simulink model "model_bicycle"  (R2024b)
settings: Solver=ode8  StartTime=0.0  StopTime=T  FixedStep=dt  MaxStep=0.01  RelTol=1e-3
values from neighbouring files (symbols this model uses):
  alpha = 10    [fcn.m]    (also in plots.m = alphas(index); plots_bicycle.m = alphas(index); plots_unicycle.m = alphas(index))
  do_filter_robot_1 = true    [plots_bicycle.m]    (also in plots_unicycle.m)
  do_filter_robot_2 = true    [plots_bicycle.m]    (also in plots_unicycle.m)
  do_probabilistic_filter = true    [plots.m]    (also in plots_bicycle.m; plots_unicycle.m)
  dt = 0.01    [plots_bicycle.m]
libraries: simulink x8, sharedTrackingLibrary x1
settings Model: Creator=maciej  LastModifiedBy=maciej

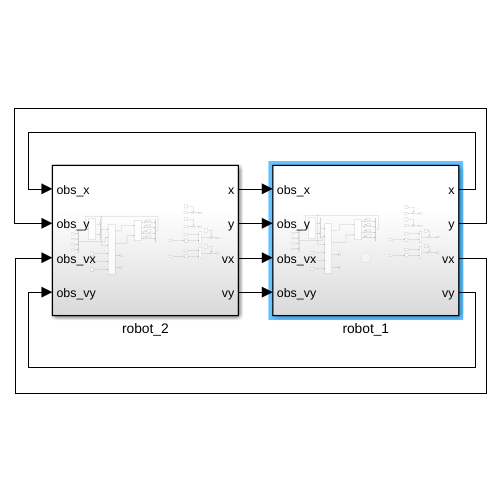
[thumbnail: Simulink's stored preview of the top-level diagram]
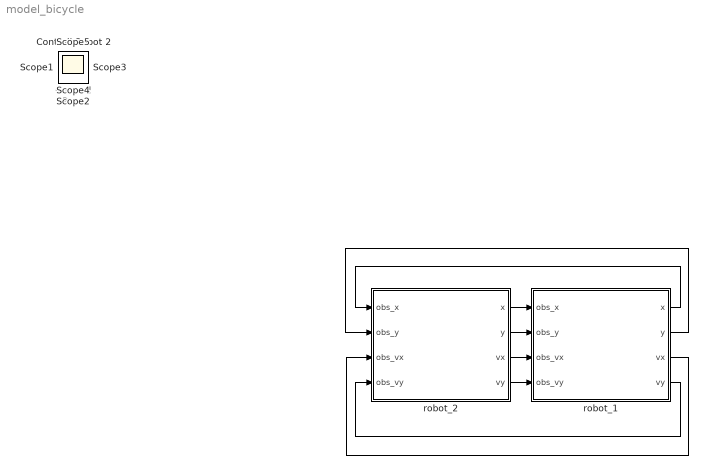
== system model_bicycle ==
  robot_1 : Subsystem
  robot_2 : Subsystem
  Controll : Scope
  Controll Robot 2 : Scope
  Pose : Scope
  Scope{,1..5} (6 alike) : Scope
  wires:
  robot_2/1(x) -> robot_1/1(obs_x)
  robot_2/2(y) -> robot_1/2(obs_y)
  robot_2/3(vx) -> robot_1/3(obs_vx)
  robot_2/4(vy) -> robot_1/4(obs_vy)
  robot_1/1(x) -> robot_2/1(obs_x)
  robot_1/2(y) -> robot_2/2(obs_y)
  robot_1/4(vy) -> robot_2/4(obs_vy)
  robot_1/3(vx) -> robot_2/3(obs_vx)

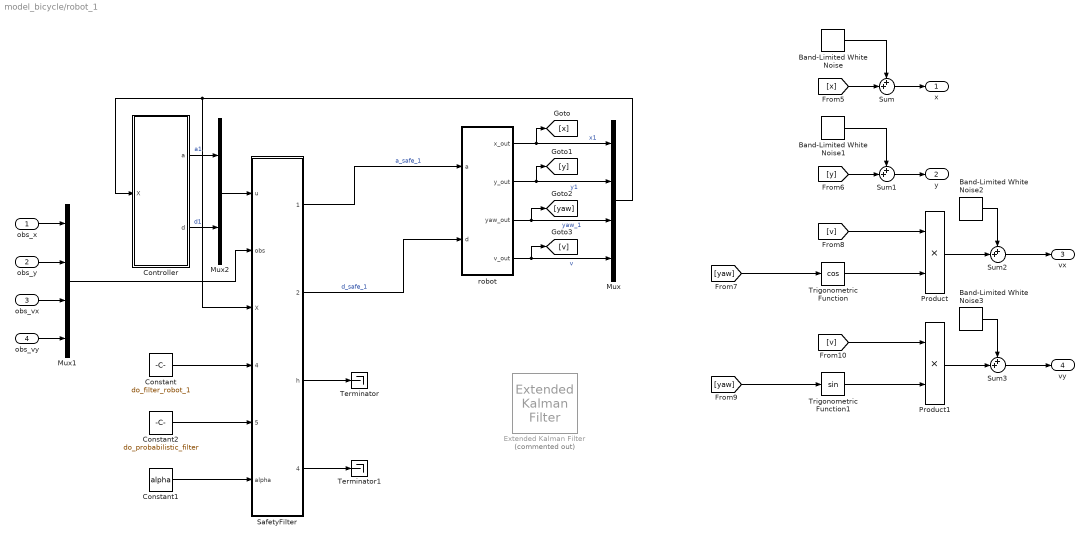
== system model_bicycle/robot_1 ==
  obs_x : Inport
  obs_y : Inport  Port=2
  obs_vx : Inport  Port=3
  obs_vy : Inport  Port=4
  Band-Limited White Noise : simulink/Sources/Band-Limited White Noise  Cov=[0.001]  Ts=dt  seed=[5]
  Band-Limited White Noise1 : simulink/Sources/Band-Limited White Noise  Cov=[0.001]  Ts=dt  seed=[6]
  Band-Limited White Noise2 : simulink/Sources/Band-Limited White Noise  Cov=[0.001]  Ts=dt  seed=[7]
  Band-Limited White Noise3 : simulink/Sources/Band-Limited White Noise  Cov=[0.001]  Ts=dt  seed=[8]
  Constant : Constant  Value=do_filter_robot_1
  Constant1 : Constant  Value=alpha
  Constant2 : Constant  Value=do_probabilistic_filter
  Controller : MATLAB Function  TreatAsAtomicUnit=on
  Extended Kalman Filter : sharedTrackingLibrary/Extended Kalman Filter  Commented=on  StateTransitionFcn=myStateTransitionFcn  HasStateTransitionJacobianFcn=off  HasAdditiveProcessNoise=Additive  ProcessNoise=1  HasTimeVaryingProcessNoise=off  HasStateTransitionFcnExtraArgument=0  InitialState=0  InitialStateCovariance=1  MeasurementFcn1=myMeasurementFcn  HasMeasurementJacobianFcn1=off  HasMeasurementEnablePort1=off  HasAdditiveMeasurementNoise1=Additive  MeasurementNoise1=[0.25 0; 0 0.25]  HasTimeVaryingMeasurementNoise1=off  HasMeasurementFcnExtraArgument1=0  HasMeasurementWrapping1=off  MeasurementFcn2=myMeasurementFcn  HasMeasurementJacobianFcn2=off  HasMeasurementEnablePort2=off  HasAdditiveMeasurementNoise2=Additive  MeasurementNoise2=1  HasTimeVaryingMeasurementNoise2=off  HasMeasurementFcnExtraArgument2=0  HasMeasurementWrapping2=off  MeasurementFcn3=myMeasurementFcn  HasMeasurementJacobianFcn3=off  HasMeasurementEnablePort3=off  HasAdditiveMeasurementNoise3=Additive  MeasurementNoise3=1  HasTimeVaryingMeasurementNoise3=off  HasMeasurementFcnExtraArgument3=0  HasMeasurementWrapping3=off  MeasurementFcn4=myMeasurementFcn  HasMeasurementJacobianFcn4=off  HasMeasurementEnablePort4=off  HasAdditiveMeasurementNoise4=Additive  MeasurementNoise4=1  HasTimeVaryingMeasurementNoise4=off  HasMeasurementFcnExtraArgument4=0  HasMeasurementWrapping4=off  MeasurementFcn5=myMeasurementFcn  HasMeasurementJacobianFcn5=off  HasMeasurementEnablePort5=off  HasAdditiveMeasurementNoise5=Additive  MeasurementNoise5=1  HasTimeVaryingMeasurementNoise5=off  HasMeasurementFcnExtraArgument5=0  HasMeasurementWrapping5=off  EnableMultirate=off  StateTransitionFcnSampleTime=1  MeasurementFcn1SampleTime=1  MeasurementFcn2SampleTime=1  MeasurementFcn3SampleTime=1  MeasurementFcn4SampleTime=1  MeasurementFcn5SampleTime=1  UseCurrentEstimator=on  OutputStateCovariance=on  DataType=double  SampleTime=-1  NumberOfMeasurements=1
  Mux : Mux
  Mux1 : Mux
  Mux2 : Mux  Inputs=2
  Product : Product
  Product1 : Product
  SafetyFilter : MATLAB Function  TreatAsAtomicUnit=on
  Sum{,1..3} (4 alike) : Sum  Inputs=++|
  Terminator : Terminator
  Terminator1 : Terminator
  Trigonometric Function : Trigonometry  Operator=cos
  Trigonometric Function1 : Trigonometry
  robot : Subsystem
  x : Outport
  y : Outport  Port=2
  vx : Outport  Port=3
  vy : Outport  Port=4
  wires:
  robot/4(v_out) -> Mux/4, [v]  "v"
  robot/3(yaw_out) -> Mux/3, [yaw]  "yaw_1"
  robot/1(x_out) -> Mux/1, [x]  "x1"
  robot/2(y_out) -> Mux/2, [y]  "y1"
  Trigonometric Function/1 -> Product/2
  [yaw] -> Trigonometric Function/1
  [v] -> Product/1
  [v] -> Product1/1
  [yaw] -> Trigonometric Function1/1
  Trigonometric Function1/1 -> Product1/2
  Mux/1 -> SafetyFilter/3(X), Controller/1(X)
  obs_x/1 -> Mux1/1
  obs_vx/1 -> Mux1/3
  obs_y/1 -> Mux1/2
  obs_vy/1 -> Mux1/4
  Controller/1(a) -> Mux2/1  "a1"
  Controller/2(d) -> Mux2/2  "d1"
  Mux2/1 -> SafetyFilter/1(u)
  Mux1/1 -> SafetyFilter/2(obs)
  SafetyFilter/1(ua_safe) -> robot/1(a)  "a_safe_1"
  SafetyFilter/2(ud_safe) -> robot/2(d)  "d_safe_1"
  SafetyFilter/3(h) -> Terminator/1
  Constant/1 -> SafetyFilter/4(do_filter)
  Band-Limited White Noise/1 -> Sum/1
  [x] -> Sum/2
  Sum/1 -> x/1
  [y] -> Sum1/2
  Sum1/1 -> y/1
  Band-Limited White Noise1/1 -> Sum1/1
  Product/1 -> Sum2/2
  Sum2/1 -> vx/1
  Product1/1 -> Sum3/2
  Sum3/1 -> vy/1
  Band-Limited White Noise2/1 -> Sum2/1
  Band-Limited White Noise3/1 -> Sum3/1
  Constant1/1 -> SafetyFilter/6(alpha)
  Constant2/1 -> SafetyFilter/5(do_probabilistic_filter)
  SafetyFilter/4(is_updated) -> Terminator1/1

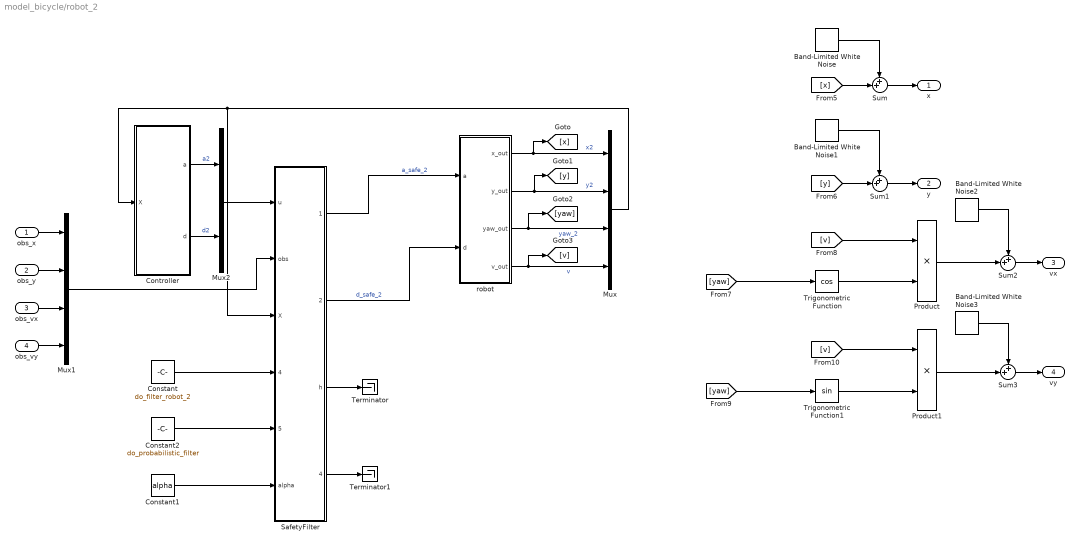
== system model_bicycle/robot_2 ==
  obs_x : Inport
  obs_y : Inport  Port=2
  obs_vx : Inport  Port=3
  obs_vy : Inport  Port=4
  Band-Limited White Noise : simulink/Sources/Band-Limited White Noise  Cov=[0.001]  Ts=dt  seed=[4]
  Band-Limited White Noise1 : simulink/Sources/Band-Limited White Noise  Cov=[0.001]  Ts=dt  seed=[3]
  Band-Limited White Noise2 : simulink/Sources/Band-Limited White Noise  Cov=[0.001]  Ts=dt  seed=[2]
  Band-Limited White Noise3 : simulink/Sources/Band-Limited White Noise  Cov=[0.001]  Ts=dt  seed=[1]
  Constant : Constant  Value=do_filter_robot_2
  Constant1 : Constant  Value=alpha
  Constant2 : Constant  Value=do_probabilistic_filter
  Controller : MATLAB Function  TreatAsAtomicUnit=on
  Mux : Mux
  Mux1 : Mux
  Mux2 : Mux  Inputs=2
  Product : Product
  Product1 : Product
  SafetyFilter : MATLAB Function  TreatAsAtomicUnit=on
  Sum{,1..3} (4 alike) : Sum  Inputs=++|
  Terminator : Terminator
  Terminator1 : Terminator
  Trigonometric Function : Trigonometry  Operator=cos
  Trigonometric Function1 : Trigonometry
  robot : Subsystem
  x : Outport
  y : Outport  Port=2
  vx : Outport  Port=3
  vy : Outport  Port=4
  wires:
  robot/4(v_out) -> Mux/4, [v]  "v"
  robot/3(yaw_out) -> Mux/3, [yaw]  "yaw_2"
  robot/1(x_out) -> Mux/1, [x]  "x2"
  robot/2(y_out) -> Mux/2, [y]  "y2"
  Trigonometric Function/1 -> Product/2
  [yaw] -> Trigonometric Function/1
  [v] -> Product/1
  [v] -> Product1/1
  [yaw] -> Trigonometric Function1/1
  Trigonometric Function1/1 -> Product1/2
  Mux/1 -> SafetyFilter/3(X), Controller/1(X)
  obs_x/1 -> Mux1/1
  obs_vx/1 -> Mux1/3
  obs_y/1 -> Mux1/2
  obs_vy/1 -> Mux1/4
  Controller/1(a) -> Mux2/1  "a2"
  Controller/2(d) -> Mux2/2  "d2"
  Mux2/1 -> SafetyFilter/1(u)
  SafetyFilter/1(ua_safe) -> robot/1(a)  "a_safe_2"
  SafetyFilter/2(ud_safe) -> robot/2(d)  "d_safe_2"
  SafetyFilter/3(h) -> Terminator/1
  Constant/1 -> SafetyFilter/4(do_filter)
  Mux1/1 -> SafetyFilter/2(obs)
  [x] -> Sum/2
  Sum/1 -> x/1
  Band-Limited White Noise/1 -> Sum/1
  [y] -> Sum1/2
  Sum1/1 -> y/1
  Band-Limited White Noise1/1 -> Sum1/1
  Sum2/1 -> vx/1
  Product/1 -> Sum2/2
  Product1/1 -> Sum3/2
  Sum3/1 -> vy/1
  Band-Limited White Noise2/1 -> Sum2/1
  Band-Limited White Noise3/1 -> Sum3/1
  Constant1/1 -> SafetyFilter/6(alpha)
  Constant2/1 -> SafetyFilter/5(do_probabilistic_filter)
  SafetyFilter/4(is_updated) -> Terminator1/1

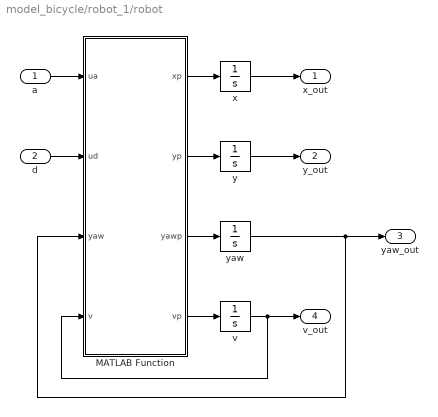
== system model_bicycle/robot_1/robot ==
  a : Inport
  d : Inport  Port=2
  MATLAB Function : MATLAB Function  TreatAsAtomicUnit=on
  v : Integrator  InitialCondition=0.01
  x : Integrator  InitialCondition=-10
  y : Integrator
  yaw : Integrator
  x_out : Outport
  y_out : Outport  Port=2
  yaw_out : Outport  Port=3
  v_out : Outport  Port=4
  wires:
  d/1 -> MATLAB Function/2(ud)
  MATLAB Function/3(yawp) -> yaw/1
  y/1 -> y_out/1
  MATLAB Function/2(yp) -> y/1
  yaw/1 -> MATLAB Function/3(yaw), yaw_out/1
  v/1 -> MATLAB Function/4(v), v_out/1
  x/1 -> x_out/1
  MATLAB Function/1(xp) -> x/1
  MATLAB Function/4(vp) -> v/1
  a/1 -> MATLAB Function/1(ua)

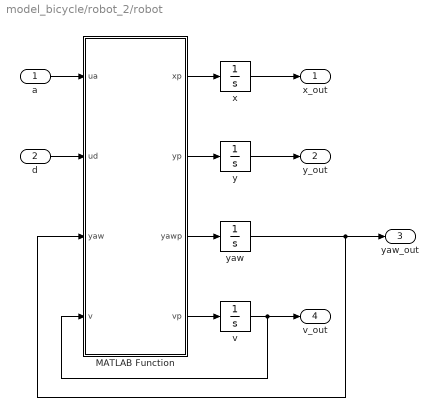
== system model_bicycle/robot_2/robot ==
  a : Inport
  d : Inport  Port=2
  MATLAB Function : MATLAB Function  TreatAsAtomicUnit=on
  v : Integrator  InitialCondition=0.01
  x : Integrator
  y : Integrator  InitialCondition=-10
  yaw : Integrator  InitialCondition=pi/2
  x_out : Outport
  y_out : Outport  Port=2
  yaw_out : Outport  Port=3
  v_out : Outport  Port=4
  wires:
  d/1 -> MATLAB Function/2(ud)
  MATLAB Function/3(yawp) -> yaw/1
  y/1 -> y_out/1
  MATLAB Function/2(yp) -> y/1
  yaw/1 -> MATLAB Function/3(yaw), yaw_out/1
  v/1 -> MATLAB Function/4(v), v_out/1
  x/1 -> x_out/1
  MATLAB Function/1(xp) -> x/1
  MATLAB Function/4(vp) -> v/1
  a/1 -> MATLAB Function/1(ua)

== matlab function model_bicycle/robot_2/Controller ==
  settings: updateMethod=DISCRETE
  data: X input; a output; d output
function [a, d] = fcn(X)
    % x_b = [x; y; theta; v]
    % x_d = [x_d; y_d; theta_d; v_d]
    % params = struct('lf',..,'lr',..,'kp_pos',..,'kp_ang',..,'kd_ang',..)
    
    % % --- Parametry ---
    lf = 1;
    lr = 1;
    kp_pos = 0.02;
    kp_ang = 3;
    kd_ang = 0.5;
    % 
    % % --- Aktualne i zadane stany ---
    x = X(1); y = X(2); theta = X(3); v = X(4);
    x_d = 0; y_d = 10; theta_d = pi/2; v_d = 0;
    % 
    % % --- Błąd pozycji ---
    ex = x_d - x;
    ey = y_d - y;
    ed = sqrt(ex^2 + ey^2);

    % --- Kierunek do celu ---
    theta_ref = atan2(ey, ex);

    % --- Błąd orientacji ---
    e_theta = wrapToPi(theta_ref - theta);

    % --- Sterowanie prędkością ---
    a_b = kp_pos * (v_d + ed - v);  % prosty regulator proporcjonalny

    % --- Sterowanie kierownicą ---
    % PD regulator na kąt
    persistent e_theta_prev
    if isempty(e_theta_prev)
        e_theta_prev = 0;
    end
    de_theta = e_theta - e_theta_prev;
    delta_b = kp_ang * e_theta + kd_ang * de_theta;
    e_theta_prev = e_theta;

    % Ograniczenie skrętu
    delta_b = max(min(delta_b, deg2rad(30)), deg2rad(-30));
    if ed < 0.1
        delta_b = 0;
    end

    % --- Wyjście ---
    a = a_b;
    d = delta_b;

    %%%%%%%%%%%%%%%%%%%%%%
    k_v = 1.0;      % do V
    k_theta = 1.0;
    c = 1.0;
    L = 2;
    v_min = 0.05;   % unikanie dzielenia przez zero

    w_a = 1.0; w_d = 10.0; w_delta = 1000;   % dobierz wagi
    H = diag([w_a, w_d, w_delta]);
    f = [0; 0; 0];

    % zx = x - x_d;
    % zy = y - y_d;
    % zt = theta - theta_d;
    % zv = v - v_d;
    ex = cos(theta)*(x - x_d) + sin(theta)*(y - y_d);   % e_x^b
    ey = -sin(theta)*(x - x_d) + cos(theta)*(y - y_d);  % e_y^b
    zt = wrapToPi(theta - theta_d);
    zv = v - v_d;


    V = 0.5*(ex^2 + ey^2 + zt^2 + zv^2);

    % a_part = zv;
    % d_part = (zt*zv) / L;
    % free_part = zv*zx*cos(zt) + zv*zy*sin(zt);
    % A = [a_part, d_part];
    % b = -free_part - 1*V;
    % 
    % 
    % options = optimoptions('quadprog', ...
    %     'Algorithm', 'active-set', ...
    %     'Display', 'off', ...
    %     'ConstraintTolerance', 1e-6, ...
    %     'OptimalityTolerance', 1e-6);
    % 
    % % solve with fallback
    % u = quadprog(H, f, A, b, [], [], [], [], [0;0], options);
    % 
    % a = u(1);
    % d = atan(u(2));

    % CLF constraint: A_clf * [a; d] <= b_clf + delta
    v_eff = max(abs(v), v_min);  % bezpieczny v
    A_clf = [ v_eff/k_v,  k_theta*zt*(v_eff/L) ];   % 1x2
    b_clf = - ex * v_eff - c * V;
    
    A = [ A_clf, -1 ];   % przenieść delta na prawą stronę: A*[a;d;delta] <= b
    b = b_clf;
    
    % bounds
    a_min = -300.0; a_max = 300.0;       % przykładowe
    d_max = 0.75; d_min = -0.75;     % rad
    lb = [a_min; d_min; 0];
    ub = [a_max; d_max; 1e6];
    
    % opcje solvera
    options = optimoptions('quadprog','Display','off','Algorithm','active-set');
    
    % solve
    [u,~,exitflag] = quadprog(H,f,A,b,[],[],lb,ub,[0;0;0],options);
    
    if exitflag <= 0
        % fallback: spróbuj bez delta albo użyj prostego regulatora P
        % tutaj prosta alternatywa:
        a = -1.0 * zv;
        d = 0;
    else
        a = -2*ex - 5*zv;%  -u(1);
        d = delta_b;%atan(u(2));
    end
end

== matlab function model_bicycle/robot_1/Controller ==
  settings: updateMethod=DISCRETE
  data: X input; a output; d output
function [a, d] = fcn(X)
    % x_b = [x; y; theta; v]
    % x_d = [x_d; y_d; theta_d; v_d]
    % params = struct('lf',..,'lr',..,'kp_pos',..,'kp_ang',..,'kd_ang',..)
    
    % % --- Parametry ---
    lf = 1;
    lr = 1;
    kp_pos = 0.02;
    kp_ang = 3;
    kd_ang = 0.5;

    % % --- Aktualne i zadane stany ---
    x = X(1); y = X(2); theta = X(3); v = X(4);
    x_d = 10; y_d = 0; theta_d = 0; v_d = 0;
    % 
    % --- Błąd pozycji ---
    ex = x_d - x;
    ey = y_d - y;
    ed = sqrt(ex^2 + ey^2);

    % --- Kierunek do celu ---
    theta_ref = atan2(ey, ex);

    % --- Błąd orientacji ---
    e_theta = wrapToPi(theta_ref - theta);

    % --- Sterowanie prędkością ---
    a_b = kp_pos * (v_d + ed - v);  % prosty regulator proporcjonalny

    % --- Sterowanie kierownicą ---
    % PD regulator na kąt
    persistent e_theta_prev
    if isempty(e_theta_prev)
        e_theta_prev = 0;
    end
    de_theta = e_theta - e_theta_prev;
    delta_b = kp_ang * e_theta + kd_ang * de_theta;
    e_theta_prev = e_theta;

    % Ograniczenie skrętu
    delta_b = max(min(delta_b, deg2rad(30)), deg2rad(-30));
    if ed < 0.1
        delta_b = 0;
    end

    % --- Wyjście ---
    a = a_b;
    d = delta_b;

    %%%%%%%%%%%%%%%%%%%
    k_v = 1.0;      % do V
    k_theta = 1.0;
    c = 0.01;
    L = 2;
    v_min = 0.05;   % unikanie dzielenia przez zero

    w_a = 1.0; w_d = 10.0; w_delta = 1000;   % dobierz wagi
    H = diag([w_a, w_d, w_delta]);
    f = [0; 0; 0];

    % zx = x - x_d;
    % zy = y - y_d;
    % zt = theta - theta_d;
    % zv = v - v_d;
    ex = cos(theta)*(x - x_d) + sin(theta)*(y - y_d);   % e_x^b
    ey = -sin(theta)*(x - x_d) + cos(theta)*(y - y_d);  % e_y^b
    zt = wrapToPi(theta - theta_d);
    zv = v - v_d;


    V = 0.5*(ex^2 + ey^2 + zt^2 + zv^2);

    % a_part = zv;
    % d_part = (zt*zv) / L;
    % free_part = zv*zx*cos(zt) + zv*zy*sin(zt);
    % A = [a_part, d_part];
    % b = -free_part - 1*V;
    % 
    % 
    % options = optimoptions('quadprog', ...
    %     'Algorithm', 'active-set', ...
    %     'Display', 'off', ...
    %     'ConstraintTolerance', 1e-6, ...
    %     'OptimalityTolerance', 1e-6);
    % 
    % % solve with fallback
    % u = quadprog(H, f, A, b, [], [], [], [], [0;0], options);
    % 
    % a = u(1);
    % d = atan(u(2));

    % CLF constraint: A_clf * [a; d] <= b_clf + delta
    v_eff = v;%max(abs(v), v_min);  % bezpieczny v
    A_clf = [ v_eff/k_v,  k_theta*zt*(v_eff/L) ];   % 1x2
    b_clf = - ex * v_eff - c * V;
    
    A = [ A_clf, -1 ];   % przenieść delta na prawą stronę: A*[a;d;delta] <= b
    b = b_clf;
    
    % bounds
    a_min = -300.0; a_max = 300.0;       % przykładowe
    d_max = 0.75; d_min = -0.75;     % rad
    lb = [a_min; d_min; 0];
    ub = [a_max; d_max; 1e6];
    
    % opcje solvera
    options = optimoptions('quadprog','Display','off','Algorithm','active-set');
    
    % solve
    [u,~,exitflag] = quadprog(H,f,A,b,[],[],lb,ub,[0;0;0],options);
    
    if exitflag <= 0
        % fallback: spróbuj bez delta albo użyj prostego regulatora P
        % tutaj prosta alternatywa:
        a = -1.0 * zv;
        d = 0;
    else
        a = -2*ex - 5 * zv;%u(1);
        d = delta_b;% atan(u(2));
    end
end

== matlab function model_bicycle/robot_1/SafetyFilter ==
  settings: updateMethod=DISCRETE
  data: u input size=2; obs input size=4; X input; ua_safe output size=1; ud_safe output size=1; h output; do_filter input; do_probabilistic_filter input; alpha input; is_updated output
function [ua_safe, ud_safe, h, is_updated] = fcn(u, obs, X, do_filter, do_probabilistic_filter, alpha)
if do_filter    
    % Parameters
    r = 1;
    lr = 0.5;
    lf = 0.5;
    L = lf + lf;
    % alpha = 1000;
    eps_safe = 1e-8;
    % control (nominal)
    ua = u(1);
    ud = tan(u(2));
    beta = atan(tan(ud) * lr / (lf + lr));
    % Obstacle
    pox = obs(1); poy = obs(2);
    vox = obs(3); voy = obs(4);
    % Host state
    xh = X(1); yh = X(2); phi = X(3); v = X(4);
    % positions / velocities / accelerations
    phx = xh; phy = yh;
    vhx = v * cos(phi + beta); vhy = v * sin(phi + beta);
    ahx = ua * cos(phi) - (v^2/lr) * ud * sin(phi);
    ahy = ua * sin(phi) + (v^2/lr) * ud * cos(phi);
    % relative
    prx = pox - phx;
    pry = poy - phy;
    vrx = vox - vhx;
    vry = voy - vhy;

    po = [pox; poy]; vo = [vox; voy];
    ph = [phx; phy]; vh = [vhx; vhy]; ah = [ahx; ahy];

    pr = po - ph; vr = vo - vh; ar = -ah;

    % bezpieczne denominatory
    vel_rel_sq = (vrx)^2 + (vry)^2;
    vel_rel_sq = max(vel_rel_sq, eps_safe);

    dist_sq = prx^2 + pry^2;
    dist = sqrt(max(dist_sq, eps_safe));
    inside_sqrt = dist_sq - r^2;
    inside_sqrt = max(inside_sqrt, 0.01);

    % S = sqrt(norm(pr)^2 - r^2)

    % Base h
    % skrócone flagi do wyrażeń
    S = sqrt(inside_sqrt);
    V2 = vel_rel_sq;
    h = pr'*vr + norm(pr)*norm(vr)*S/norm(pr);

    % Wyprowadzone części
    a_part = cos(phi)*(phx - pox) - ((cos(phi)*(vox - v*cos(phi)) + sin(phi)*(voy - v*sin(phi)))*(- r^2 + abs(phx - pox)^2 + abs(phy - poy)^2)^(1/2))/(abs(vox - v*cos(phi))^2 + abs(voy - v*sin(phi))^2) + sin(phi)*(phy - poy);
    d_part = (((v^2*sin(phi)*(vox - v*cos(phi)))/L - (v^2*cos(phi)*(voy - v*sin(phi)))/L)*(- r^2 + abs(phx - pox)^2 + abs(phy - poy)^2)^(1/2))/(abs(vox - v*cos(phi))^2 + abs(voy - v*sin(phi))^2) + (v^2*cos(phi)*(phy - poy))/L - (v^2*sin(phi)*(phx - pox))/L;
    free_part = (vox - v*cos(phi))^2 + (voy - v*sin(phi))^2 - (((vox - v*cos(phi))*(phx - pox) + (voy - v*sin(phi))*(phy - poy))*(abs(vox - v*cos(phi))^2 + abs(voy - v*sin(phi))^2))/(- r^2 + abs(phx - pox)^2 + abs(phy - poy)^2)^(1/2);

    % Macierze do QP: A*u <= b
    A = [a_part, d_part];
    b = -free_part - alpha * h;

    % QP: min 1/2 (u-u_nom)'*H*(u-u_nom)  => H, f = -H*u_nom
    w_a = 1; w_d = 1;
    H = 0.5 * diag([w_a, w_d]);
    f = -H * u;

    % For robust
    if (norm(pr)^2 - r^2) > 0 
        delta = sqrt(norm(pr)^2 - r^2);
    else
        delta = 0.01;
    end

    if do_probabilistic_filter
        nabla_p_h = vr + (norm(vr) / delta)*pr;
        nabla_v_h = pr + (delta / norm(vr))*vr;
    
        nabla_p_h_prim = ar + (vr'*ar / norm(vr) / delta)*pr + (norm(vr) / delta)*vr - (norm(vr)*pr'*vr/delta^3)*pr;
        nabla_v_h_prim = 2*vr + delta * (ar/norm(vr) - (vr'*ar/norm(vr)^3)*vr) + (norm(vr)*pr + (pr'*vr/norm(vr))*vr) / delta;
        nabla_a_h_prim = pr + (delta/norm(vr))*vr;
    
        cov_p = 0.2^2;
        cov_v = 0.2^2;
        cov_a = 0.2^2;
    
        nabla_p = nabla_p_h_prim + nabla_p_h;
        nabla_v = nabla_v_h_prim + nabla_v_h;
        nabla_a = nabla_a_h_prim;
    
        cov_c = nabla_p'*cov_p*nabla_p +  nabla_v'*cov_v*nabla_v + nabla_a'*cov_a*nabla_a;
        sigma_c = sqrt(cov_c);
    
        b = b + norminv(0.95) * sigma_c;
    end

    % bounds
    lb = [];
    ub = [];

    options = optimoptions('quadprog', ...
        'Algorithm', 'active-set', ...
        'Display', 'off', ...
        'ConstraintTolerance', 1e-6, ...
        'OptimalityTolerance', 1e-6);

    % solve with fallback
    u_safe = quadprog(H, f, -A, -b, [], [], lb, ub, u, options);
    if isempty(u_safe) || any(isnan(u_safe))
        u_safe = u;
    end

    if all(u_safe == u)
        is_updated = false;
    else
        is_updated = true;
    end

    ua_safe = u_safe(1);
    ud_safe = atan(u_safe(2));
else
    ua_safe = u(1);
    ud_safe = u(2);
    h = 0;
    is_updated = false;
end
end

== matlab function model_bicycle/robot_2/SafetyFilter ==
  settings: updateMethod=DISCRETE
  data: u input size=2; obs input size=4; X input; ua_safe output size=1; ud_safe output size=1; h output; do_filter input; do_probabilistic_filter input; alpha input; is_updated output
function [ua_safe, ud_safe, h, is_updated] = fcn(u, obs, X, do_filter, do_probabilistic_filter, alpha)
if do_filter    
    % Parameters
    r = 1;
    lr = 0.5;
    lf = 0.5;
    L = lf + lf;
    % alpha = 1000;
    eps_safe = 1e-8;
    % control (nominal)
    ua = u(1);
    ud = tan(u(2));
    beta = atan(tan(ud) * lr / (lf + lr));
    % Obstacle
    pox = obs(1); poy = obs(2);
    vox = obs(3); voy = obs(4);
    % Host state
    xh = X(1); yh = X(2); phi = X(3); v = X(4);
    % positions / velocities / accelerations
    phx = xh; phy = yh;
    vhx = v * cos(phi + beta); vhy = v * sin(phi + beta);
    ahx = ua * cos(phi) - (v^2/lr) * ud * sin(phi);
    ahy = ua * sin(phi) + (v^2/lr) * ud * cos(phi);
    % relative
    prx = pox - phx;
    pry = poy - phy;
    vrx = vox - vhx;
    vry = voy - vhy;

    po = [pox; poy]; vo = [vox; voy];
    ph = [phx; phy]; vh = [vhx; vhy]; ah = [ahx; ahy];

    pr = po - ph; vr = vo - vh; ar = -ah;

    % bezpieczne denominatory
    vel_rel_sq = (vrx)^2 + (vry)^2;
    vel_rel_sq = max(vel_rel_sq, eps_safe);

    dist_sq = prx^2 + pry^2;
    dist = sqrt(max(dist_sq, eps_safe));
    inside_sqrt = dist_sq - r^2;
    inside_sqrt = max(inside_sqrt, 0.01);

    % S = sqrt(norm(pr)^2 - r^2)

    % Base h
    % skrócone flagi do wyrażeń
    S = sqrt(inside_sqrt);
    V2 = vel_rel_sq;
    h = pr'*vr + norm(pr)*norm(vr)*S/norm(pr);

    % Wyprowadzone części
    a_part = cos(phi)*(phx - pox) - ((cos(phi)*(vox - v*cos(phi)) + sin(phi)*(voy - v*sin(phi)))*(- r^2 + abs(phx - pox)^2 + abs(phy - poy)^2)^(1/2))/(abs(vox - v*cos(phi))^2 + abs(voy - v*sin(phi))^2) + sin(phi)*(phy - poy);
    d_part = (((v^2*sin(phi)*(vox - v*cos(phi)))/L - (v^2*cos(phi)*(voy - v*sin(phi)))/L)*(- r^2 + abs(phx - pox)^2 + abs(phy - poy)^2)^(1/2))/(abs(vox - v*cos(phi))^2 + abs(voy - v*sin(phi))^2) + (v^2*cos(phi)*(phy - poy))/L - (v^2*sin(phi)*(phx - pox))/L;
    free_part = (vox - v*cos(phi))^2 + (voy - v*sin(phi))^2 - (((vox - v*cos(phi))*(phx - pox) + (voy - v*sin(phi))*(phy - poy))*(abs(vox - v*cos(phi))^2 + abs(voy - v*sin(phi))^2))/(- r^2 + abs(phx - pox)^2 + abs(phy - poy)^2)^(1/2);

    % Macierze do QP: A*u <= b
    A = [a_part, d_part];
    b = -free_part - alpha * h;

    % QP: min 1/2 (u-u_nom)'*H*(u-u_nom)  => H, f = -H*u_nom
    w_a = 1; w_d = 1;
    H = 0.5 * diag([w_a, w_d]);
    f = - H * u;

    % For robust
    if (norm(pr)^2 - r^2) > 0 
        delta = sqrt(norm(pr)^2 - r^2);
    else
        delta = 0.01;
    end

    if do_probabilistic_filter
        nabla_p_h = vr + (norm(vr) / delta)*pr;
        nabla_v_h = pr + (delta / norm(vr))*vr;
    
        nabla_p_h_prim = ar + (vr'*ar / norm(vr) / delta)*pr + (norm(vr) / delta)*vr - (norm(vr)*pr'*vr/delta^3)*pr;
        nabla_v_h_prim = 2*vr + delta * (ar/norm(vr) - (vr'*ar/norm(vr)^3)*vr) + (norm(vr)*pr + (pr'*vr/norm(vr))*vr) / delta;
        nabla_a_h_prim = pr + (delta/norm(vr))*vr;
    
        cov_p = 0.2^2;
        cov_v = 0.2^2;
        cov_a = 0.2^2;
    
        nabla_p = nabla_p_h_prim + nabla_p_h;
        nabla_v = nabla_v_h_prim + nabla_v_h;
        nabla_a = nabla_a_h_prim;
    
        cov_c = nabla_p'*cov_p*nabla_p +  nabla_v'*cov_v*nabla_v + nabla_a'*cov_a*nabla_a;
        sigma_c = sqrt(cov_c);
    
        b = b + norminv(0.99) * sigma_c;
    end

    % bounds
    lb = [];
    ub = [];

    options = optimoptions('quadprog', ...
        'Algorithm', 'active-set', ...
        'Display', 'off', ...
        'ConstraintTolerance', 1e-6, ...
        'OptimalityTolerance', 1e-6);

    % solve with fallback
    u_safe = quadprog(H, f, -A, -b, [], [], lb, ub, u, options);
    if isempty(u_safe) || any(isnan(u_safe))
        u_safe = u;
    end

    if all(u_safe == u)
        is_updated = false;
    else
        is_updated = true;
    end

    ua_safe = u_safe(1);
    ud_safe = atan(u_safe(2));
else
    ua_safe = u(1);
    ud_safe = u(2);
    h = 0;
    is_updated = false;
end
end

== matlab function model_bicycle/robot_1/robot/MATLAB Function ==
  data: ua input; xp output; ud input; yaw input; v input; yp output; yawp output; vp output
function [xp, yp, yawp, vp] = fcn(ua, ud, yaw, v)
    lr = 1;
    lf = 1;

    xp = v * cos(yaw);
    yp = v * sin(yaw);
    yawp = (v/lr) * tan(ud);
    vp = ua;

end

== matlab function model_bicycle/robot_2/robot/MATLAB Function ==
  data: ua input; xp output; ud input; yaw input; v input; yp output; yawp output; vp output
function [xp, yp, yawp, vp] = fcn(ua, ud, yaw, v)
    lr = 1;
    lf = 1;

    beta = atan((lr / (lr + lf)) * tan(ud));

    xp = v * cos(yaw + beta);
    yp = v * sin(yaw + beta);
    yawp = (v/lr) * sin(beta);
    vp = ua;

end
